simulink model "Kalman"  (R2020b)
settings: Solver=VariableStepAuto  StartTime=0.0  StopTime=10.0  RelTol=1e-3
values from neighbouring files (symbols this model uses):
  A = [0 0;1 0]    [KalmanParameters.m]
  B = [1/J;0]    [KalmanParameters.m]
  b = 0.5    [KalmanParameters.m]
  C = zeros(2,2)    [KalmanParameters.m]
  D = zeros(2,3)    [KalmanParameters.m]
  initial = [10,10]    [KalmanParameters.m]
  InitialK = [0,0.1]    [KalmanParameters.m]
  J = 6689.281*10^-6    (= 0.006689281)    [KalmanParameters.m]
  Ko = Ko'    [KalmanParameters.m]
  kp = 0.4    [KalmanParameters.m]
  L = 284.84*10^-3    (= 0.28484)    [KalmanParameters.m]
  n = 1/100    (= 0.01)    [KalmanParameters.m]
  PWMs_fixed = [1619,1638]    [KalmanParameters.m]
  Td = 0.5780    (= 0.578)    [KalmanParameters.m]
  Ti = 1.1    [KalmanParameters.m]
undefined symbols (not defined in the file or in its folder): sigbuilder_block
libraries: pid_lib x1
settings Model: Creator=lorem  LastModifiedBy=lorem

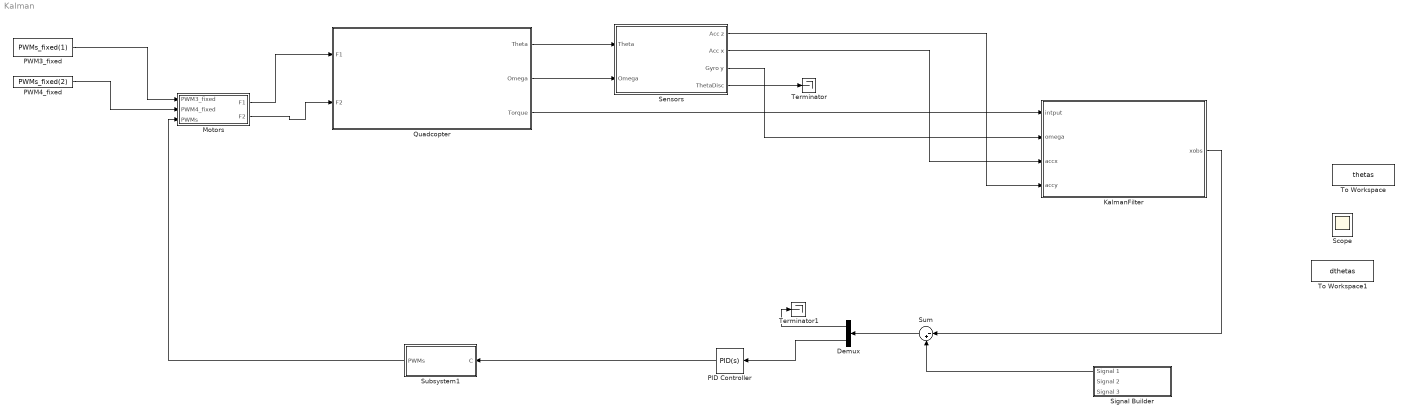
== system Kalman ==
  Demux : Demux  Outputs=2
  KalmanFilter : Subsystem
  Motors : Subsystem
  PID Controller : pid_lib/PID Controller  Controller=PID  Form=Parallel  TimeDomain=Continuous-time  UseExternalTs=off  SampleTime=-1  IntegratorMethod=Forward Euler  FilterMethod=Forward Euler  ControllerParametersSource=internal  P=kp  I=kp/Ti  D=kp*Td  UseFilter=on  N=1/n  TunerSelectOption=Transfer Function Based (PID Tuner App)  InitialConditionSource=internal  InitialConditionForIntegrator=0  InitialConditionForFilter=0  DifferentiatorICPrevScaledInput=0  ExternalReset=none  TrackingMode=off  Kt=1  LimitOutput=off  SatLimitsSource=internal  UpperSaturationLimit=inf  LowerSaturationLimit=-inf  LinearizeAsGain=on  AntiWindupMode=none  Kb=1  POutMin=[]  POutMax=[]  IOutMin=[]  IOutMax=[]  DOutMin=[]  DOutMax=[]  NOutMin=[]  NOutMax=[]  SumOutMin=[]  SumOutMax=[]  SaturationOutMin=[]  SaturationOutMax=[]  PParamMin=[]  PParamMax=[]  IParamMin=[]  IParamMax=[]  DParamMin=[]  DParamMax=[]  NParamMin=[]  NParamMax=[]  KbParamMin=[]  KbParamMax=[]  KtParamMin=[]  KtParamMax=[]  KbOutMin=[]  KbOutMax=[]  KtOutMin=[]  KtOutMax=[]  IntegratorOutMin=[]  IntegratorOutMax=[]  FilterOutMin=[]  FilterOutMax=[]  SumI1OutMin=[]  SumI1OutMax=[]  SumI2OutMin=[]  SumI2OutMax=[]  SumI3OutMin=[]  SumI3OutMax=[]  SumI4OutMin=[]  SumI4OutMax=[]  SumDOutMin=[]  SumDOutMax=[]  DifferentiatorOutMin=[]  DifferentiatorOutMax=[]  FilterDiffOutCoefMin=[]  FilterDiffOutCoefMax=[]  ReciprocalOutMin=[]  ReciprocalOutMax=[]  SumDenOutMin=[]  SumDenOutMax=[]  SumNumOutMin=[]  SumNumOutMax=[]  DivideOutMin=[]  DivideOutMax=[]  UdiffTsProdOutMin=[]  UdiffTsProdOutMax=[]  NTsProdOutMin=[]  NTsProdOutMax=[]  UintegralTsProdOutMin=[]  UintegralTsProdOutMax=[]  UngainTsProdOutMin=[]  UngainTsProdOutMax=[]  IntegratorContinuousStateAttributes=''  IntegratorStateMustResolveToSignalObject=off  IntegratorRTWStateStorageClass=Auto  FilterContinuousStateAttributes=''  FilterStateMustResolveToSignalObject=off  FilterRTWStateStorageClass=Auto  ParallelPVariant=InternalParameters  IdealPVariant=Disabled  IVariant=InternalParameters  DVariant=InternalParameters  IntegratorVariant=Continuous  SatVariant=Disabled  AWVariant=Passthrough  PCopyVariant=Disabled  TRVariant=Disabled  FdbkBlocksVariant=Forward  IdealPFdbkVariant=Disabled  SatFdbkVariant=Disabled  DerivativeFilterVariant=ContFilter  NVariant=InternalParameters  NCopyVariant=Disabled  FilterICVariant=InternalICsFilter  IntegratorICVariant=InternalICs  ExternalResetVariant=Disabled  TRSumVariant=Passthrough  SumFdbkVariant=Disabled  SumVariant=Sum_PID  TsampFilterVariant=InternalTs  TsampNgainVariant=Passthrough  TsampIntegralVariant=Passthrough  ExternalSaturationOutDataTypeStr=Inherit: Same as second input
  PWM3_fixed : Constant  Value=PWMs_fixed(1)  SampleTime=0.02
  PWM4_fixed : Constant  Value=PWMs_fixed(2)  SampleTime=0.02
  Quadcopter : Subsystem
  Scope : Scope  NumInputPorts=2
  Sensors : Subsystem
  Signal Builder : Subsystem  Tag=STV Subsys  LoadFcn=sigbuilder_block('load');  StartFcn=sigbuilder_block('start');  StopFcn=sigbuilder_block('stop');  ClipboardFcn=sigbuilder_block('clipboard');  mask(Sigbuilder block){tuvar=[0:10]}
      mask help: Simulink:masks:SigbuilderBlock_MD
      mask init:
      | if ~strcmp(get_param(bdroot(gcbh),'SimulationStatus'),'stopped') tuvar = sigbuilder_block('maskInit'); end
      settings: CopyFcn=sigbuilder_block('copy');  DeleteFcn=sigbuilder_block('delete');  ModelCloseFcn=sigbuilder_block('modelClose');  PreSaveFcn=sigbuilder_block('preSave');  PauseFcn=sigbuilder_block('pause');  ContinueFcn=sigbuilder_block('continue');  NameChangeFcn=sigbuilder_block('namechange');  OpenFcn=sigbuilder_block('open',[6.75 6.75 1138.5 568.5 ]);  CloseFcn=sigbuilder_block('close');
      mask Display: plot(0, 0, 100, 100,[2, 2, 32, 32, 2], [68, 8, 8, 68, 68],[32, 2], [38, 38], [32, 19, 2],[53, 60, 44], [32, 17, 17, 2],[16, 16, 31, 31]);txt = getActiveGroup(gcbh);text(2, 100, txt,'verticalAlignment', 'top');
  Subsystem1 : Subsystem
  Sum : Sum  Inputs=|-+
  Terminator : Terminator
  Terminator1 : Terminator
  To Workspace : ToWorkspace  VariableName=thetas  SaveFormat=Timeseries  SampleTime=-1
  To Workspace1 : ToWorkspace  VariableName=dthetas  SaveFormat=Timeseries  SampleTime=-1
  wires:
  Sensors/4(ThetaDisc) -> Terminator/1
  Quadcopter/2(Omega) -> Sensors/2(Omega)
  Quadcopter/1(Theta) -> Sensors/1(Theta)
  PWM4_fixed/1 -> Motors/2(PWM4_fixed)
  Motors/2(F2) -> Quadcopter/2(F2)
  PWM3_fixed/1 -> Motors/1(PWM3_fixed)
  Motors/1(F1) -> Quadcopter/1(F1)
  Subsystem1/1(PWMs) -> Motors/3(PWMs)
  Signal Builder/1(Signal 1) -> Sum/2
  PID Controller/1 -> Subsystem1/1(C)
  Sum/1 -> Demux/1
  Demux/2 -> PID Controller/1
  Demux/1 -> Terminator1/1
  Quadcopter/3("Torque ") -> KalmanFilter/1(intput)
  Sensors/3(Gyro y) -> KalmanFilter/2(omega)
  Sensors/2(Acc x) -> KalmanFilter/3(accx)
  Sensors/1(Acc z) -> KalmanFilter/4(accy)
  KalmanFilter/1(xobs) -> Sum/1

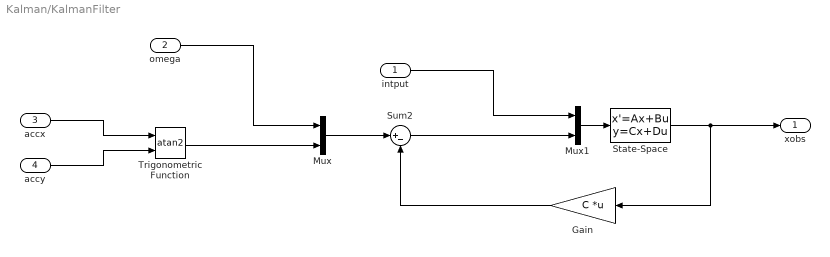
== system Kalman/KalmanFilter ==
  intput : Inport
  omega : Inport  Port=2
  accx : Inport  Port=3
  accy : Inport  Port=4
  Gain : Gain  Gain=C  Multiplication=Matrix(K*u) (u vector)
  Mux : Mux  Inputs=2
  Mux1 : Mux  Inputs=2
  State-Space : StateSpace  A=A  B=[B Ko]  C=eye(2,2)  D=D  InitialCondition=InitialK
  Sum2 : Sum  Inputs=|+-
  Trigonometric Function : Trigonometry  Operator=atan2
  xobs : Outport
  wires:
  Trigonometric Function/1 -> Mux/2
  Gain/1 -> Sum2/2
  Mux1/1 -> State-Space/1
  State-Space/1 -> xobs/1, Gain/1
  Sum2/1 -> Mux1/2
  intput/1 -> Mux1/1
  Mux/1 -> Sum2/1
  omega/1 -> Mux/1
  accy/1 -> Trigonometric Function/2
  accx/1 -> Trigonometric Function/1

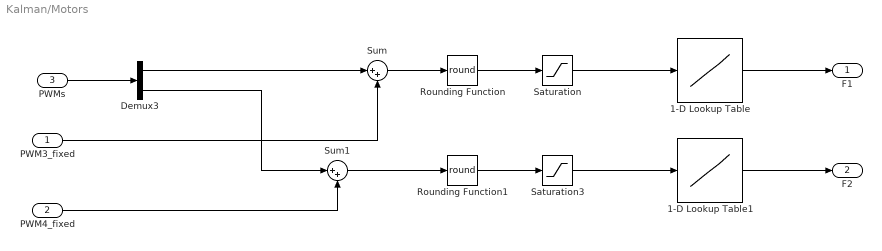
== system Kalman/Motors ==
  PWM3_fixed : Inport
  PWM4_fixed : Inport  Port=2
  PWMs : Inport  Port=3
  1-D Lookup Table : Lookup_n-D  NumberOfTableDimensions=1  BreakpointsForDimension1=[1447,1792]  Table=[1.1,4.8]  InternalRulePriority=Speed  RndMeth=Simplest  InputSameDT=on
  1-D Lookup Table1 : Lookup_n-D  NumberOfTableDimensions=1  BreakpointsForDimension1=[1455,1832]  Table=[0.9,5.2]  InternalRulePriority=Speed  RndMeth=Simplest  InputSameDT=on
  Demux3 : Demux  Outputs=2
  Rounding Function : Rounding  Operator=round
  Rounding Function1 : Rounding  Operator=round
  Saturation : Saturate  UpperLimit=1792  LowerLimit=1447
  Saturation3 : Saturate  UpperLimit=1832  LowerLimit=1455
  Sum : Sum  Inputs=|++
  Sum1 : Sum  Inputs=|++
  F1 : Outport  VectorParamsAs1DForOutWhenUnconnected=off
  F2 : Outport  Port=2  VectorParamsAs1DForOutWhenUnconnected=off
  wires:
  PWMs/1 -> Demux3/1
  PWM4_fixed/1 -> Sum1/2
  PWM3_fixed/1 -> Sum/2
  Demux3/1 -> Sum/1
  Demux3/2 -> Sum1/1
  Sum1/1 -> Rounding Function1/1
  Rounding Function1/1 -> Saturation3/1
  Sum/1 -> Rounding Function/1
  Rounding Function/1 -> Saturation/1
  Saturation/1 -> 1-D Lookup Table/1
  Saturation3/1 -> 1-D Lookup Table1/1
  1-D Lookup Table1/1 -> F2/1
  1-D Lookup Table/1 -> F1/1

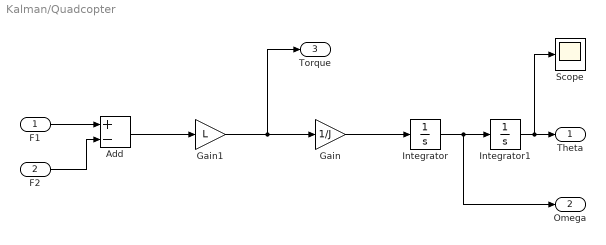
== system Kalman/Quadcopter ==
  F1 : Inport
  F2 : Inport  Port=2
  Add : Sum  Inputs=+-
  Gain : Gain  Gain=1/J
  Gain1 : Gain  Gain=L
  Integrator : Integrator  InitialCondition=deg2rad(initial(1))
  Integrator1 : Integrator  InitialCondition=deg2rad(initial(2))
  Scope : Scope
  Theta : Outport  VectorParamsAs1DForOutWhenUnconnected=off
  Omega : Outport  Port=2  VectorParamsAs1DForOutWhenUnconnected=off
  "Torque " : Outport  Port=3  VectorParamsAs1DForOutWhenUnconnected=off
  wires:
  Gain/1 -> Integrator/1
  Integrator/1 -> Omega/1, Integrator1/1
  F2/1 -> Add/2
  F1/1 -> Add/1
  Add/1 -> Gain1/1
  Gain1/1 -> "Torque "/1, Gain/1
  Integrator1/1 -> Scope/1, Theta/1

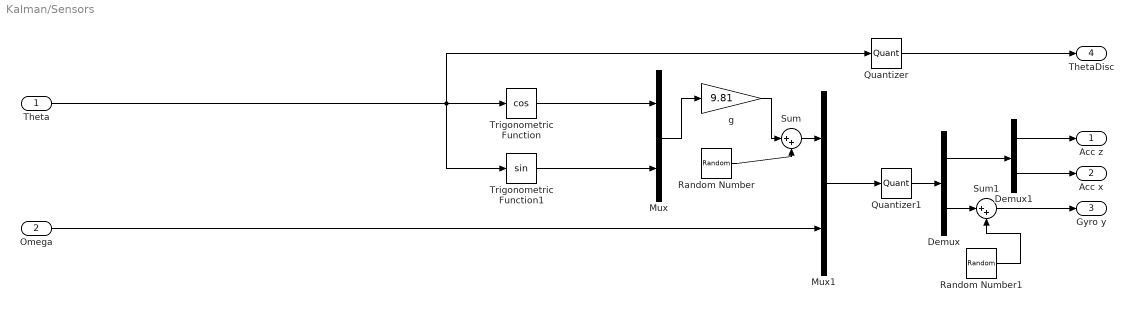
== system Kalman/Sensors ==
  Theta : Inport
  Omega : Inport  Port=2
  Demux : Demux  Outputs=2
  Demux1 : Demux  Outputs=2
  Mux : Mux  Inputs=2
  Mux1 : Mux  Inputs=2
  Quantizer : Quantizer  QuantizationInterval=0.01  SampleTime=0.02
  Quantizer1 : Quantizer  QuantizationInterval=0.01  SampleTime=0.02
  Random Number : RandomNumber  Variance=0.0127  SampleTime=0
  Random Number1 : RandomNumber  Variance=0.00127  Seed=1  SampleTime=0
  Sum : Sum  Inputs=|++
  Sum1 : Sum  Inputs=|++
  Trigonometric Function : Trigonometry  Operator=cos
  Trigonometric Function1 : Trigonometry
  g : Gain  Gain=9.81
  Acc z : Outport  VectorParamsAs1DForOutWhenUnconnected=off
  Acc x : Outport  Port=2  VectorParamsAs1DForOutWhenUnconnected=off
  Gyro y : Outport  Port=3  VectorParamsAs1DForOutWhenUnconnected=off
  ThetaDisc : Outport  Port=4  VectorParamsAs1DForOutWhenUnconnected=off
  wires:
  Trigonometric Function1/1 -> Mux/2
  Trigonometric Function/1 -> Mux/1
  Mux/1 -> g/1
  Mux1/1 -> Quantizer1/1
  Quantizer1/1 -> Demux/1
  Demux/1 -> Demux1/1
  Demux1/1 -> Acc z/1
  Omega/1 -> Mux1/2
  Theta/1 -> Quantizer/1, Trigonometric Function1/1, Trigonometric Function/1
  Demux1/2 -> Acc x/1
  Quantizer/1 -> ThetaDisc/1
  g/1 -> Sum/1
  Random Number/1 -> Sum/2
  Sum/1 -> Mux1/1
  Demux/2 -> Sum1/1
  Sum1/1 -> Gyro y/1
  Random Number1/1 -> Sum1/2

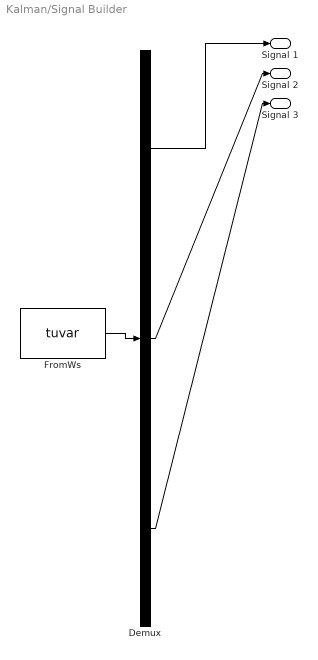
== system Kalman/Signal Builder ==
  Demux : Demux  Tag=STV Demux  Outputs=3
      settings: DisplayOption=none
  FromWs : FromWorkspace  Tag=STV FromWs  VariableName=tuvar
      SigBuilderData=|
      | common.afterFinalStr = 'Extrapolate'
      | common.sampleTime = 0
      | dataSet.timeRange = [0 10]
      | dataSet.name = 'Group 1'
      | sbobj.Groups.Name = 'Group 1'
      | sbobj.Groups.Signals(1).Name = 'Signal 1'
      | sbobj.Groups.Signals(1).XData = [0 10]
      | sbobj.Groups.Signals(1).YData = [0 0]
      | sbobj.Groups.Signals(2).Name = 'Signal 2'
      | sbobj.Groups.Signals(2).XData = [0 5 5 10]
      | sbobj.Groups.Signals(2).YData = [0 0 1 1]
      | sbobj.Groups.Signals(3).Name = 'Signal 3'
      | sbobj.Groups.Signals(3).XData = [0 5 5.001 7 7 10]
      | sbobj.Groups.Signals(3).YData = [0 0 1 1 0 0]
  Signal 1 : Outport  Tag=STV Outport  VectorParamsAs1DForOutWhenUnconnected=off
  Signal 2 : Outport  Tag=STV Outport  Port=2  VectorParamsAs1DForOutWhenUnconnected=off
  Signal 3 : Outport  Tag=STV Outport  Port=3  VectorParamsAs1DForOutWhenUnconnected=off
  wires:
  Demux/1 -> Signal 1/1
  FromWs/1 -> Demux/1
  Demux/2 -> Signal 2/1
  Demux/3 -> Signal 3/1

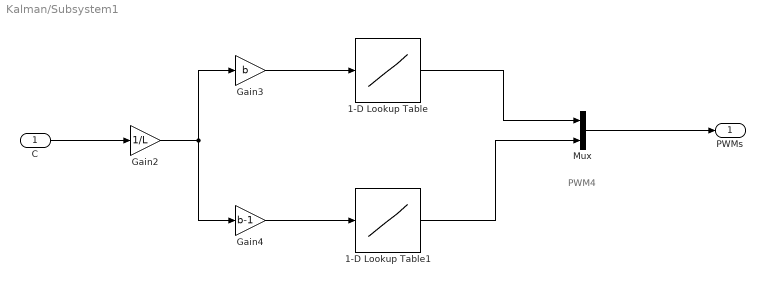
== system Kalman/Subsystem1 ==
  note: PWM4
  C : Inport
  1-D Lookup Table : Lookup_n-D  NumberOfTableDimensions=1  BreakpointsForDimension1=[-2,2]  Table=[-138,138]  InternalRulePriority=Speed  RndMeth=Simplest  InputSameDT=on
  1-D Lookup Table1 : Lookup_n-D  NumberOfTableDimensions=1  BreakpointsForDimension1=[-2,2]  Table=[-150.8,150.8]  InternalRulePriority=Speed  RndMeth=Simplest  InputSameDT=on
  Gain2 : Gain  Gain=1/L
  Gain3 : Gain  Gain=b
  Gain4 : Gain  Gain=b-1
  Mux : Mux  Inputs=2
  PWMs : Outport  VectorParamsAs1DForOutWhenUnconnected=off
  wires:
  1-D Lookup Table1/1 -> Mux/2
  Gain2/1 -> Gain3/1, Gain4/1
  1-D Lookup Table/1 -> Mux/1
  Gain4/1 -> 1-D Lookup Table1/1
  Gain3/1 -> 1-D Lookup Table/1
  Mux/1 -> PWMs/1
  C/1 -> Gain2/1
